simulink model "C_Nonlinear_alg_transform_6T"  (R2016b)
settings: Solver=ode15s  StartTime=0.0  StopTime=100  RelTol=0.01  AbsTol=0.01
libraries: dspinverses x1
settings Model: Creator=Utente  LastModifiedBy=liana
settings SolverCC: MaxOrder=3  MaxConsecutiveMinStep=5  SolverJacobianMethodControl=FullAnalytical  ZeroCrossControl=DisableAll  SolverResetMethod=Robust
settings DataIOCC: SaveState=on
settings OptimizationCC: BlockReduction=off  DefaultParameterBehavior=Inlined  BufferReuse=off

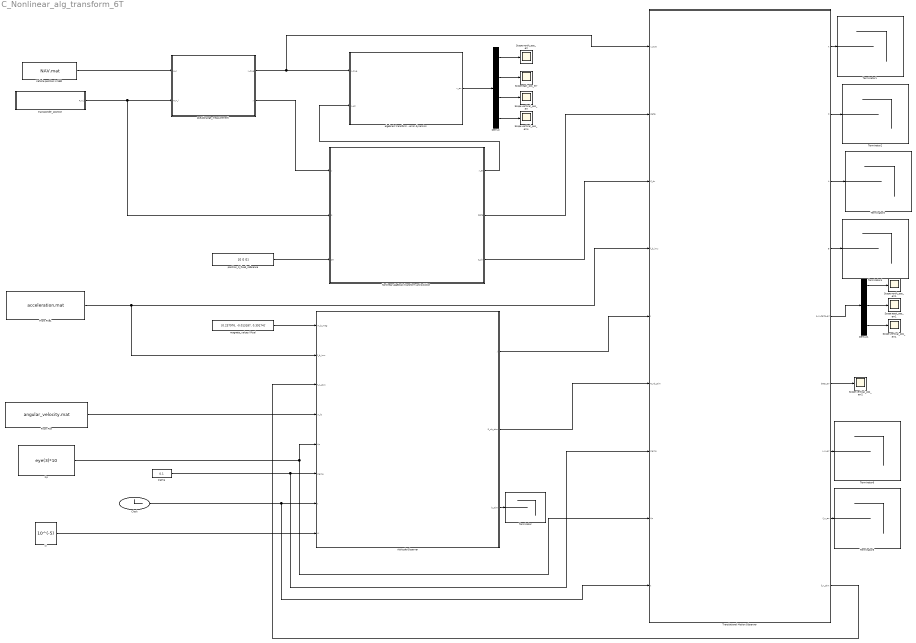
== system C_Nonlinear_alg_transform_6T ==
  Attitude Observer : Subsystem
  Clock : Clock
      settings: Decimation=50
  Demux : Demux
  Demux1 : Demux  Outputs=3
  From File : FromFile  FileName=angular_velocity.mat  SampleTime=0
  From File1 : FromFile  FileName=acceleration.mat  SampleTime=0
  Kp : Constant  Value=eye(3)*10
  Nonlinear algebraic transform and solution : Subsystem
  Scope east_pos_err : Scope
  Scope east_pos_err1 : Scope
  Scope north_pos_err : Scope
  Scope north_pos_err1 : Scope
  Scope vertical_pos_err{,1..2,4} (4 alike) : Scope
  Terminator{,1..6} (7 alike) : Terminator
  Translational Motion Observer : Subsystem
  Vehicle position in NED : FromFile  FileName=NAV.mat
  algebraic transform - error dynamics : Subsystem
  ki : Constant  Value=10^(-5)
  magneto_values (Pisa) : Constant  Value=[0.237976, -0.013187, 0.39174]'
  position_0_fixed_reference : Constant  Value=[0 0 0]
  "pseudorange_measurement " : Subsystem
  sigma : Constant  Value=0.1
  transponder_position : Subsystem
  wires:
  Demux/1 -> Scope north_pos_err/1
  Demux/2 -> Scope east_pos_err/1
  Demux/3 -> Scope vertical_pos_err/1
  Nonlinear algebraic transform and solution/1(x_at) -> algebraic transform - error dynamics/2(x_at)
  Demux/4 -> Scope vertical_pos_err4/1
  position_0_fixed_reference/1 -> Nonlinear algebraic transform and solution/3(p0)
  Nonlinear algebraic transform and solution/2(delta) -> Translational Motion Observer/2(delta)
  Nonlinear algebraic transform and solution/3(C_dx) -> Translational Motion Observer/3(C_dx)
  Vehicle position in NED/1 -> "pseudorange_measurement "/1(p_n)
  "pseudorange_measurement "/2("y ") -> Nonlinear algebraic transform and solution/1(y)
  algebraic transform - error dynamics/1(x_err) -> Demux/1
  transponder_position/1(p_n_i) -> Nonlinear algebraic transform and solution/2(p), "pseudorange_measurement "/2(p_n_i)
  magneto_values (Pisa)/1 -> Attitude Observer/1(m_b_mag)
  Translational Motion Observer/9(f_n_stim) -> Attitude Observer/3(f_n_stim)
  Attitude Observer/1(J) -> Translational Motion Observer/5(J)
  Attitude Observer/2(R_nb_stim) -> Translational Motion Observer/6(R_nb_stim)
  From File1/1 -> Attitude Observer/2(f_b_imu), Translational Motion Observer/4(f_b_imu)
  Kp/1 -> Attitude Observer/5(Kp), Translational Motion Observer/8(Kp)
  sigma/1 -> Translational Motion Observer/7(sigma), Attitude Observer/6(sigma)
  ki/1 -> Attitude Observer/8(Ki)
  Clock/1 -> Translational Motion Observer/9(t), Attitude Observer/7(t)
  From File/1 -> Attitude Observer/4(w_ib)
  Attitude Observer/3(b_stim) -> Terminator/1
  "pseudorange_measurement "/1(x_true) -> Translational Motion Observer/1(x_true), algebraic transform - error dynamics/1(x_true)
  Translational Motion Observer/1(K) -> Terminator1/1
  Translational Motion Observer/2("C ") -> Terminator2/1
  Translational Motion Observer/3(" A") -> Terminator3/1
  Translational Motion Observer/4(B) -> Terminator4/1
  Translational Motion Observer/8(f_n_err) -> Terminator5/1
  Translational Motion Observer/7(v_n_err) -> Terminator6/1
  Demux1/1 -> Scope north_pos_err1/1
  Demux1/2 -> Scope east_pos_err1/1
  Demux1/3 -> Scope vertical_pos_err1/1
  Translational Motion Observer/6(beta_err) -> Scope vertical_pos_err2/1
  Translational Motion Observer/5(p_n_delta_err) -> Demux1/1

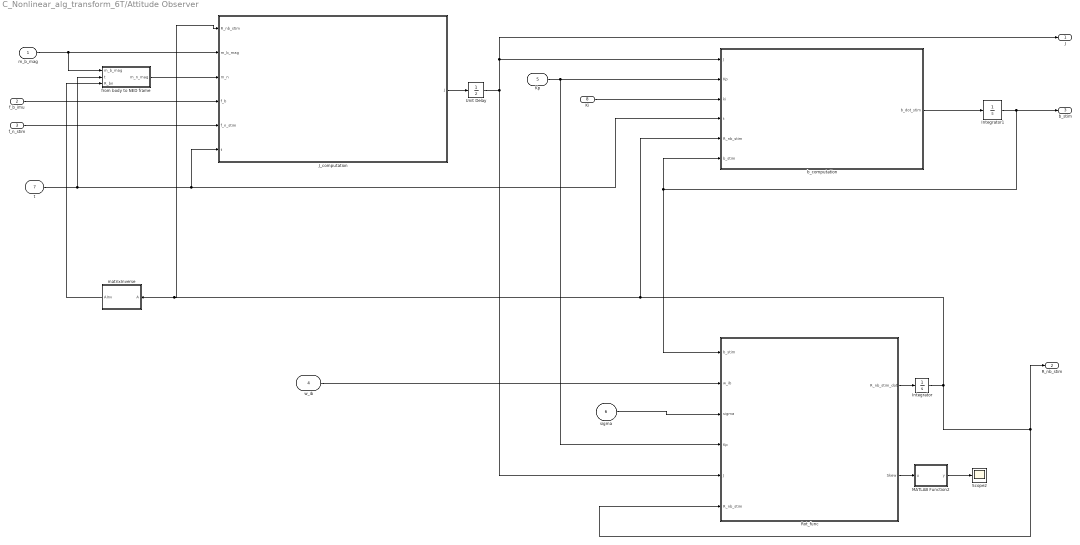
== system C_Nonlinear_alg_transform_6T/Attitude Observer ==
  m_b_mag : Inport
  f_b_imu : Inport  Port=2
  f_n_stim : Inport  Port=3
  w_ib : Inport  Port=4
  Kp : Inport  Port=5
  sigma : Inport  Port=6
  t : Inport  Port=7
  Ki : Inport  Port=8
  Integrator : Integrator  InitialCondition=eye(3)  AbsoluteTolerance=0.0000000001
  Integrator1 : Integrator  InitialCondition=0.02  UpperSaturationLimit=100  LowerSaturationLimit=-100  AbsoluteTolerance=0.0000001
  J_computation : Subsystem
  MATLAB Function2 : MATLAB Function  TreatAsAtomicUnit=on
  Rot_func : MATLAB Function  TreatAsAtomicUnit=on
  Scope2 : Scope
  Unit Delay : UnitDelay  SampleTime=-1
  b_computation : MATLAB Function  TreatAsAtomicUnit=on
  from body to NED frame : MATLAB Function  TreatAsAtomicUnit=on
  matrixInverse : MATLAB Function  TreatAsAtomicUnit=on
  J : Outport
  R_nb_stim : Outport  Port=2
  b_stim : Outport  Port=3
  wires:
  m_b_mag/1 -> from body to NED frame/1(m_b_mag), J_computation/2(m_b_mag)
  from body to NED frame/1(m_n_mag) -> J_computation/3(m_n)
  f_b_imu/1 -> J_computation/4(f_b)
  Kp/1 -> Rot_func/4(Kp), b_computation/2(Kp)
  Ki/1 -> b_computation/3(ki)
  sigma/1 -> Rot_func/3(sigma)
  w_ib/1 -> Rot_func/2(w_ib)
  t/1 -> from body to NED frame/2(t), b_computation/4(t), J_computation/6(t)
  b_computation/1(b_dot_stim) -> Integrator1/1
  matrixInverse/1(AInv) -> from body to NED frame/3(R_bn)
  MATLAB Function2/1(y) -> Scope2/1
  Rot_func/2(Skew) -> MATLAB Function2/1(u)
  Rot_func/1(R_nb_stim_dot) -> Integrator/1
  f_n_stim/1 -> J_computation/5(f_n_stim)
  Integrator/1 -> J_computation/1(R_nb_stim), matrixInverse/1(A), b_computation/5(R_nb_stim), Rot_func/6(R_nb_stim), R_nb_stim/1
  Integrator1/1 -> Rot_func/1(b_stim), b_computation/6(b_stim), b_stim/1
  J_computation/1(J) -> Unit Delay/1
  Unit Delay/1 -> b_computation/1(J), J/1, Rot_func/5(J)

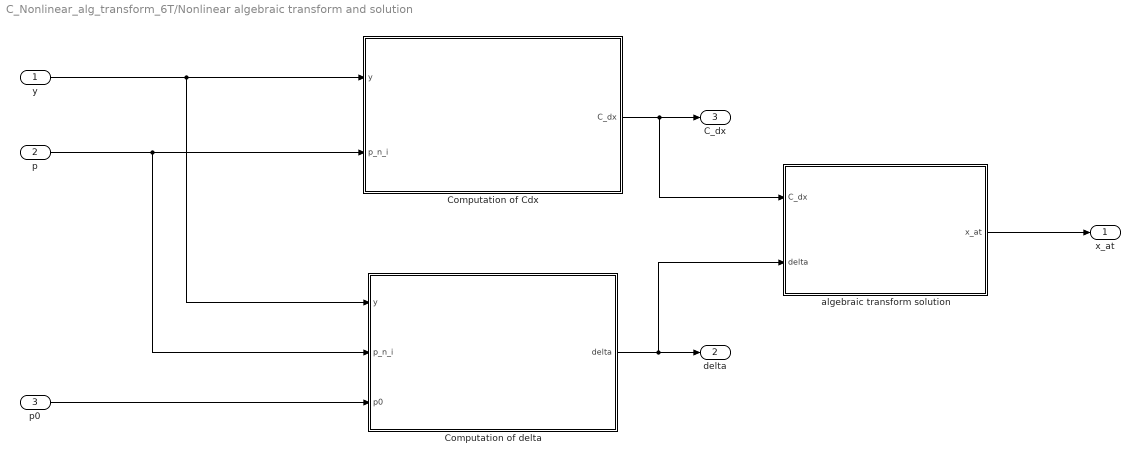
== system C_Nonlinear_alg_transform_6T/Nonlinear algebraic transform and solution ==
  y : Inport
  p : Inport  Port=2
  p0 : Inport  Port=3
  Computation of Cdx : MATLAB Function  TreatAsAtomicUnit=on
  Computation of delta : MATLAB Function  TreatAsAtomicUnit=on
  algebraic transform solution : MATLAB Function  TreatAsAtomicUnit=on
  x_at : Outport
  delta : Outport  Port=2
  C_dx : Outport  Port=3
  wires:
  y/1 -> Computation of delta/1(y), Computation of Cdx/1(y)
  p/1 -> Computation of delta/2(p_n_i), Computation of Cdx/2(p_n_i)
  p0/1 -> Computation of delta/3(p0)
  Computation of delta/1(delta) -> algebraic transform solution/2(delta), delta/1
  Computation of Cdx/1(C_dx) -> algebraic transform solution/1(C_dx), C_dx/1
  algebraic transform solution/1(x_at) -> x_at/1

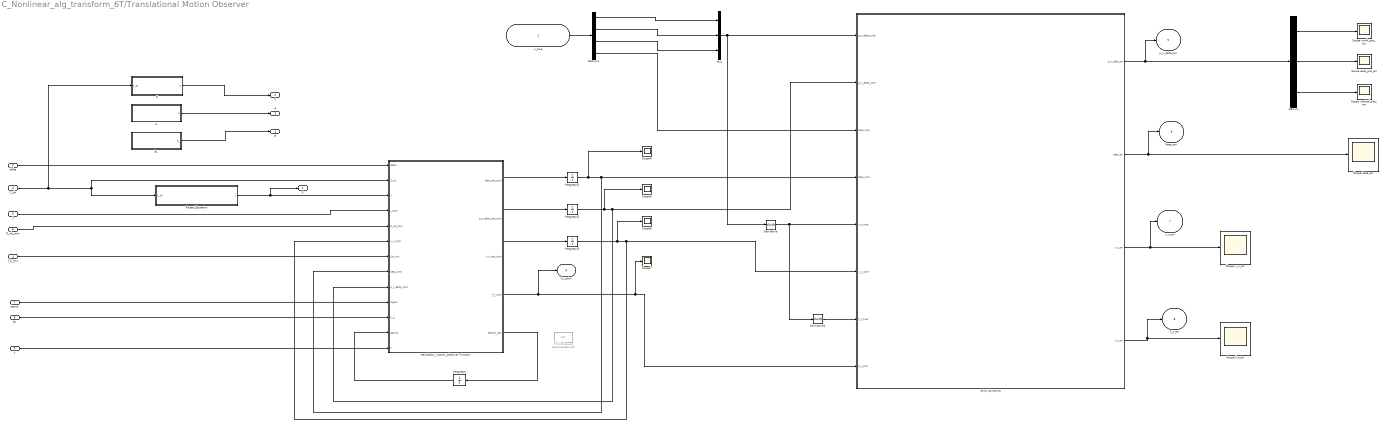
== system C_Nonlinear_alg_transform_6T/Translational Motion Observer ==
  x_true : Inport
  delta : Inport  Port=2
  C_dx : Inport  Port=3
  f_b_imu : Inport  Port=4
  J : Inport  Port=5
  R_nb_stim : Inport  Port=6
  sigma : Inport  Port=7
  Kp : Inport  Port=8
  t : Inport  Port=9
  A : MATLAB Function  TreatAsAtomicUnit=on
  B_ : MATLAB Function  TreatAsAtomicUnit=on
  C : MATLAB Function  TreatAsAtomicUnit=on
  Demux : Demux  Outputs=3
  Demux1 : Demux
  Derivative : Derivative
  Derivative1 : Derivative
  Integrator : Integrator  AbsoluteTolerance=0.01
  Integrator1 : Integrator  InitialCondition=100  AbsoluteTolerance=0.00001
  Integrator2 : Integrator  AbsoluteTolerance=0.01
  Integrator3 : Integrator  AbsoluteTolerance=0.01
  Mux : Mux  Inputs=3
  Riccati_Equation : Subsystem
  Scope beta_err : Scope
  Scope f_n_err : Scope
  Scope v_n_err : Scope
  Scope east_pos_err : Scope
  Scope north_pos_err : Scope
  Scope vertical_pos_err : Scope
  Scope{4..7} (4 alike) : Scope
  To Workspace : ToWorkspace  Commented=on  VariableName=KO  SaveFormat=Timeseries  SampleTime=-1
  error dynamics : MATLAB Function  TreatAsAtomicUnit=on
  translation_motion_observer Function : MATLAB Function  TreatAsAtomicUnit=on
  K : Outport
  "C " : Outport  Port=2
  " A" : Outport  Port=3
  B : Outport  Port=4
  p_n_delta_err : Outport  Port=5
  beta_err : Outport  Port=6
  v_n_err : Outport  Port=7
  f_n_err : Outport  Port=8
  f_n_stim : Outport  Port=9
  wires:
  translation_motion_observer Function/4(f_n_stim) -> f_n_stim/1, Scope7/1, error dynamics/8(f_n_stim)
  translation_motion_observer Function/3(v_n_dot_stim) -> Integrator3/1
  translation_motion_observer Function/2(p_n_delta_dot_stim) -> Integrator2/1
  C_dx/1 -> C/1(C_dx), Riccati_Equation/1(C_dx), translation_motion_observer Function/2(C_dx)
  J/1 -> translation_motion_observer Function/4(J_stim)
  R_nb_stim/1 -> translation_motion_observer Function/5(R_nb_stim)
  delta/1 -> translation_motion_observer Function/1(delta)
  f_b_imu/1 -> translation_motion_observer Function/7(f_b_imu)
  sigma/1 -> translation_motion_observer Function/10(sigma)
  Kp/1 -> translation_motion_observer Function/11(K_p)
  A/1(A) -> " A"/1
  C/1(C) -> "C "/1
  Riccati_Equation/1(K) -> K/1, translation_motion_observer Function/3(K)
  B_/1(B_) -> B/1
  t/1 -> translation_motion_observer Function/13(t)
  Integrator3/1 -> Scope6/1, error dynamics/6(v_n_stim), translation_motion_observer Function/6(v_n_stim)
  translation_motion_observer Function/1(beta_dot_stim) -> Integrator1/1
  Integrator/1 -> translation_motion_observer Function/12(epsilon)
  Integrator1/1 -> Scope4/1, translation_motion_observer Function/8(beta_stim), error dynamics/4(beta_stim)
  translation_motion_observer Function/5(epsilon_dot) -> Integrator/1
  Integrator2/1 -> Scope5/1, error dynamics/2(p_n_delta_stim), translation_motion_observer Function/9(p_n_delta_stim)
  Mux/1 -> Derivative/1, error dynamics/1(p_n_delta_true)
  Demux1/4 -> error dynamics/3(beta_true)
  Derivative1/1 -> error dynamics/7(f_n_true)
  error dynamics/2(beta_err) -> beta_err/1, Scope beta_err/1
  error dynamics/4(f_n_err) -> f_n_err/1, Scope f_n_err/1
  error dynamics/3(v_n_err) -> v_n_err/1, Scope v_n_err/1
  error dynamics/1(p_n_delta_err) -> Demux/1, p_n_delta_err/1
  Demux/1 -> Scope north_pos_err/1
  Demux/2 -> Scope east_pos_err/1
  Demux/3 -> Scope vertical_pos_err/1
  x_true/1 -> Demux1/1
  Demux1/3 -> Mux/3
  Demux1/2 -> Mux/2
  Demux1/1 -> Mux/1
  Derivative/1 -> Derivative1/1, error dynamics/5(v_n_true)

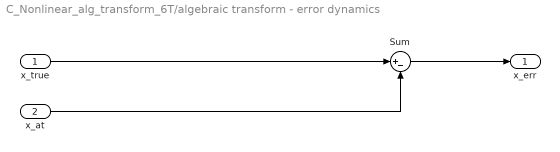
== system C_Nonlinear_alg_transform_6T/algebraic transform - error dynamics ==
  x_true : Inport
  x_at : Inport  Port=2
  Sum : Sum  Inputs=|+-
  x_err : Outport
  wires:
  x_at/1 -> Sum/2
  Sum/1 -> x_err/1
  x_true/1 -> Sum/1

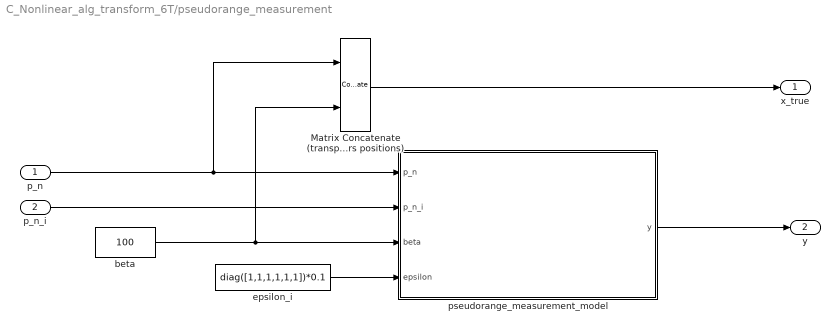
== system C_Nonlinear_alg_transform_6T/pseudorange_measurement  ==
  p_n : Inport
  p_n_i : Inport  Port=2
  Matrix Concatenate (transponders positions) : Concatenate  Mode=Multidimensional array
  beta : Constant  Value=100
  epsilon_i : Constant  Value=diag([1,1,1,1,1,1])*0.1
  pseudorange_measurement_model : MATLAB Function  TreatAsAtomicUnit=on
  x_true : Outport
  "y " : Outport  Port=2
  wires:
  p_n_i/1 -> pseudorange_measurement_model/2(p_n_i)
  pseudorange_measurement_model/1(y) -> "y "/1
  epsilon_i/1 -> pseudorange_measurement_model/4(epsilon)
  beta/1 -> Matrix Concatenate (transponders positions)/2, pseudorange_measurement_model/3(beta)
  p_n/1 -> Matrix Concatenate (transponders positions)/1, pseudorange_measurement_model/1(p_n)
  Matrix Concatenate (transponders positions)/1 -> x_true/1

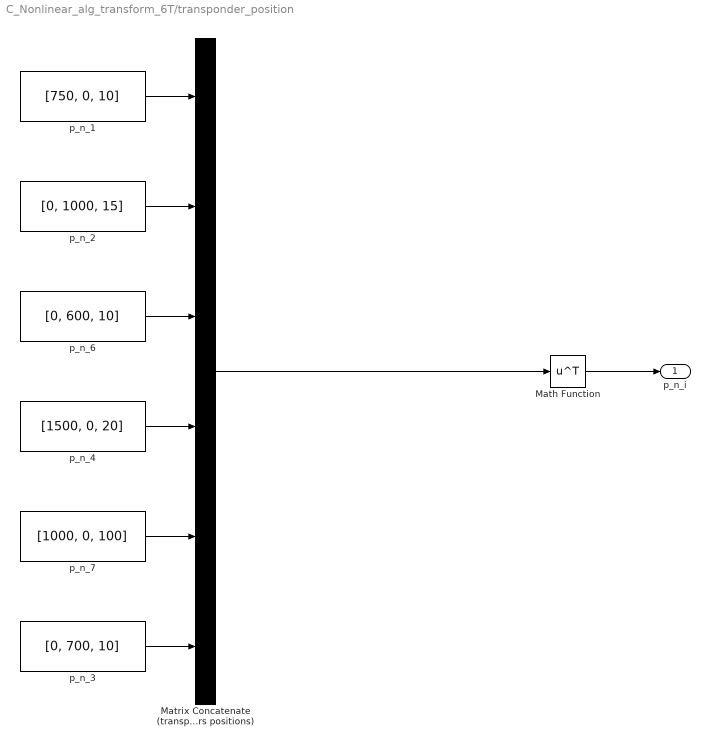
== system C_Nonlinear_alg_transform_6T/transponder_position ==
  Math Function : Math  Operator=transpose  SaturateOnIntegerOverflow=on
  Matrix Concatenate (transponders positions) : Concatenate  NumInputs=6  Mode=Multidimensional array  ConcatenateDimension=2
  p_n_1 : Constant  Value=[750, 0, 10]
  p_n_2 : Constant  Value=[0, 1000, 15]
  p_n_3 : Constant  Value=[0, 700, 10]
  p_n_4 : Constant  Value=[1500, 0, 20]
  p_n_6 : Constant  Value=[0, 600, 10]
  p_n_7 : Constant  Value=[1000, 0, 100]
  p_n_i : Outport
  wires:
  Matrix Concatenate (transponders positions)/1 -> Math Function/1
  p_n_4/1 -> Matrix Concatenate (transponders positions)/4
  p_n_7/1 -> Matrix Concatenate (transponders positions)/5
  p_n_3/1 -> Matrix Concatenate (transponders positions)/6
  Math Function/1 -> p_n_i/1
  p_n_1/1 -> Matrix Concatenate (transponders positions)/1
  p_n_2/1 -> Matrix Concatenate (transponders positions)/2
  p_n_6/1 -> Matrix Concatenate (transponders positions)/3

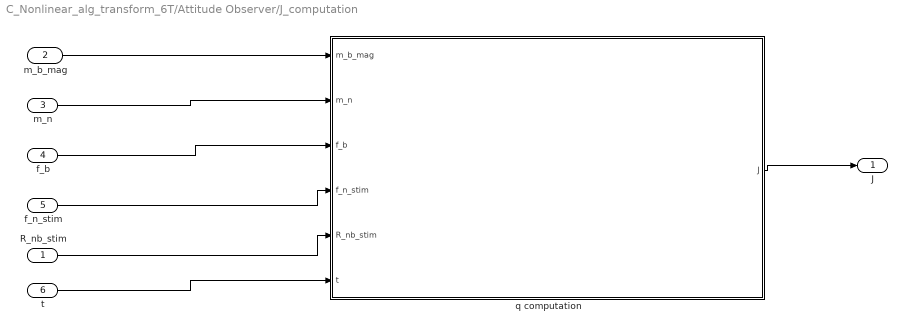
== system C_Nonlinear_alg_transform_6T/Attitude Observer/J_computation ==
  R_nb_stim : Inport
  m_b_mag : Inport  Port=2
  m_n : Inport  Port=3
  f_b : Inport  Port=4
  f_n_stim : Inport  Port=5
  t : Inport  Port=6
  q computation : MATLAB Function  TreatAsAtomicUnit=on
  J : Outport
  wires:
  m_n/1 -> q computation/2(m_n)
  f_n_stim/1 -> q computation/4(f_n_stim)
  m_b_mag/1 -> q computation/1(m_b_mag)
  f_b/1 -> q computation/3(f_b)
  q computation/1(J) -> J/1
  R_nb_stim/1 -> q computation/5(R_nb_stim)
  t/1 -> q computation/6(t)

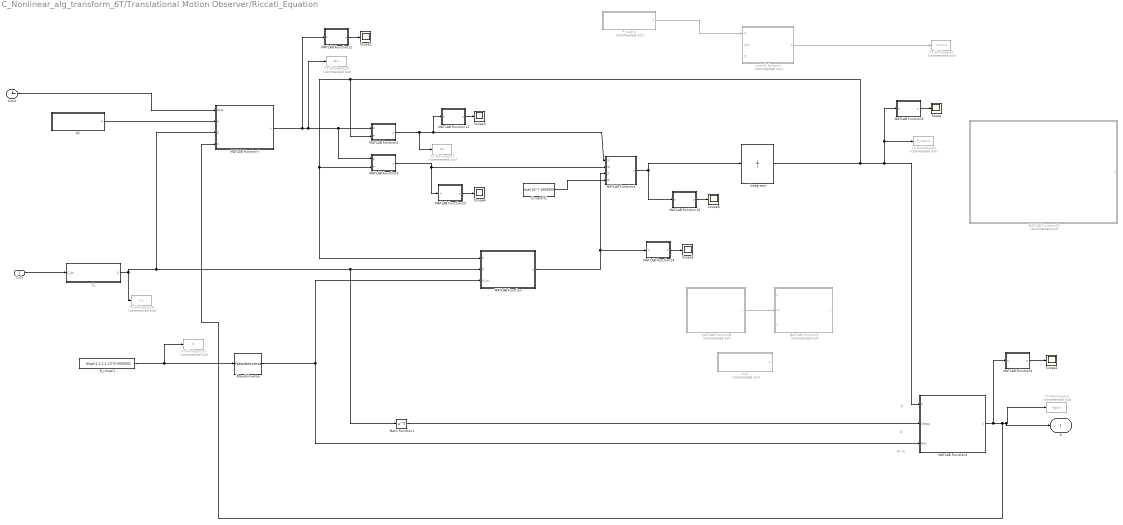
== system C_Nonlinear_alg_transform_6T/Translational Motion Observer/Riccati_Equation ==
  note: R^-1
  note: C'
  note: P
  C_dx : Inport
  A1 : MATLAB Function  TreatAsAtomicUnit=on
  C_ : MATLAB Function  TreatAsAtomicUnit=on
  Clock : Clock
  Integrator : Integrator  InitialCondition=eye(10)*10  AbsoluteTolerance=0.000001
  MATLAB Function : MATLAB Function  TreatAsAtomicUnit=on
  MATLAB Function1 : MATLAB Function  TreatAsAtomicUnit=on
  MATLAB Function10 : MATLAB Function  Commented=on  TreatAsAtomicUnit=on
  MATLAB Function11 : MATLAB Function  TreatAsAtomicUnit=on
  MATLAB Function12 : MATLAB Function  TreatAsAtomicUnit=on
  MATLAB Function13 : MATLAB Function  TreatAsAtomicUnit=on
  MATLAB Function14 : MATLAB Function  TreatAsAtomicUnit=on
  MATLAB Function16 : MATLAB Function  TreatAsAtomicUnit=on
  MATLAB Function2 : MATLAB Function  TreatAsAtomicUnit=on
  MATLAB Function3 : MATLAB Function  TreatAsAtomicUnit=on
  MATLAB Function4 : MATLAB Function  TreatAsAtomicUnit=on
  MATLAB Function5 : MATLAB Function  TreatAsAtomicUnit=on
  MATLAB Function6 : MATLAB Function  TreatAsAtomicUnit=on
  MATLAB Function7 : MATLAB Function  TreatAsAtomicUnit=on
  MATLAB Function8 : MATLAB Function  Commented=on  TreatAsAtomicUnit=on
  MATLAB Function9 : MATLAB Function  Commented=on  TreatAsAtomicUnit=on
  Math Function1 : Math  Operator=transpose  SaturateOnIntegerOverflow=on
  "P_matrix " : MATLAB Function  Commented=on  TreatAsAtomicUnit=on
  Pseudoinverse : dspinverses/Pseudoinverse  wanterr=off  SimulateUsing=Interpreted execution
  Q matrix1 : Constant  Value=eye(10) * 1000000
  R_riccati1 : Constant  Value=diag([1,1,1,1,1])*0.0000001  VectorParams1D=off
  Scope{,1..6} (7 alike) : Scope
  To Workspace1 : ToWorkspace  Commented=on  VariableName=P_matrix  SampleTime=-1
  To Workspace2 : ToWorkspace  Commented=on  VariableName=simout  SaveFormat=Timeseries  SampleTime=-1
  To Workspace3 : ToWorkspace  Commented=on  VariableName=Kgain  SaveFormat=Timeseries  SampleTime=-1
  To Workspace5 : ToWorkspace  Commented=on  VariableName=R  SaveFormat=Timeseries  SampleTime=-1
  To Workspace7 : ToWorkspace  Commented=on  VariableName=PA  SaveFormat=Timeseries  SampleTime=-1
  To Workspace8 : ToWorkspace  Commented=on  VariableName=C_n  SaveFormat=Timeseries  SampleTime=-1
  To Workspace9 : ToWorkspace  Commented=on  VariableName=AKC  SaveFormat=Timeseries  SampleTime=-1
  myC : MATLAB Function  Commented=on  TreatAsAtomicUnit=on
  switch_function : MATLAB Function  Commented=on  TreatAsAtomicUnit=on
  K : Outport
  wires:
  R_riccati1/1 -> Pseudoinverse/1, To Workspace5/1
  Math Function1/1 -> MATLAB Function4/2(Ctrasp)
  MATLAB Function2/1(y) -> To Workspace7/1, MATLAB Function12/1(u), MATLAB Function1/1(X)
  MATLAB Function3/1(y) -> MATLAB Function13/1(u), MATLAB Function1/2(W)
  MATLAB Function/1(y) -> MATLAB Function14/1(u), MATLAB Function1/3(Z)
  MATLAB Function1/1(y) -> Integrator/1, MATLAB Function16/1(u)
  C_dx/1 -> C_/1(C_dx)
  Clock/1 -> MATLAB Function7/1(clock)
  "P_matrix "/1(P) -> switch_function/1(P1)
  switch_function/1(P) -> To Workspace2/1
  Integrator/1 -> MATLAB Function4/1(P), MATLAB Function5/1(u), To Workspace1/1, MATLAB Function2/2(P), MATLAB Function3/2(P), MATLAB Function/1(P)
  MATLAB Function5/1(y) -> Scope/1
  MATLAB Function6/1(y) -> Scope1/1
  MATLAB Function8/1(y) -> MATLAB Function9/2(CK)
  MATLAB Function4/1(y) -> MATLAB Function6/1(u), MATLAB Function7/4(K), K/1, To Workspace3/1
  A1/1(A) -> MATLAB Function7/2(A)
  C_/1(C) -> To Workspace8/1, MATLAB Function7/3(C), Math Function1/1, MATLAB Function/2(C)
  MATLAB Function7/1(y) -> MATLAB Function11/1(u), To Workspace9/1, MATLAB Function3/1(A), MATLAB Function2/1(A)
  MATLAB Function11/1(y) -> Scope2/1
  MATLAB Function12/1(y) -> Scope3/1
  MATLAB Function13/1(y) -> Scope4/1
  MATLAB Function14/1(y) -> Scope5/1
  Pseudoinverse/1 -> MATLAB Function4/3(Rinv), MATLAB Function/3(R_inv)
  MATLAB Function16/1(y) -> Scope6/1
  Q matrix1/1 -> MATLAB Function1/4(Q)

== matlab function C_Nonlinear_alg_transform_6T/Translational Motion Observer/Riccati_Equation/MATLAB Function ==
  data: P input; y output; C input; R_inv input
function y = fcn(P,C,R_inv)

y = - P * C' * R_inv * C * P;

end

== matlab function C_Nonlinear_alg_transform_6T/Attitude Observer/J_computation/q computation ==
  data: m_b_mag input; m_n input; f_b input; f_n_stim input size=3; J output; R_nb_stim input size=[3,3]; t input
function J  = qEfunc(m_b_mag, m_n, f_b, f_n_stim, R_nb_stim, t)

% if t <= 1
%     R_nb_stim = eye(3);
% end

g_n = [0.1 0.1 9.81]';

q1_b = m_b_mag/norm(m_b_mag,2);
q2_b = f_b/norm(g_n,2);

q1_n = m_n/norm(m_n,2);
q2_n = f_n_stim/norm(g_n,2);


E_b = [q1_b, skew(q1_b)*q2_b, (skew(q1_b)*skew(q1_b))*q2_b];
E_n = [q1_n, skew(q1_n)*q2_n, (skew(q1_n)*skew(q1_n))*q2_n];

J = (E_n - R_nb_stim * E_b) * (E_b');

end

== matlab function C_Nonlinear_alg_transform_6T/Translational Motion Observer/Riccati_Equation/MATLAB Function1 ==
  data: X input; y output size=[10,10]; W input; Z input; Q input
function y = fcn(X,W,Z,Q)

y =  X + W + Z + Q;
% y = Z + Q;

end

== matlab function C_Nonlinear_alg_transform_6T/Translational Motion Observer/Riccati_Equation/A1 ==
  data: A output
function A = A()

 A = zeros(10);

A(1:3,5:7) = eye(3);
A(5:7,8:10) = eye(3);
 

% A = eye(10);

end

== matlab function C_Nonlinear_alg_transform_6T/Attitude Observer/b_computation ==
  data: J input; b_dot_stim output size=3; Kp input; ki input; t input; R_nb_stim input; b_stim input
function b_dot_stim  = b_dot_stim_func(J, Kp, ki, t, R_nb_stim, b_stim)


%b_dot_stim = zeros(3 ,1);

% if t <= 1
%     R_nb_stim = eye(3);
% %      b_stim = zeros(3, 1);
% %     
% end

SAT = sat(R_nb_stim)';
PA = pa( SAT * Kp * J);
VEX = vexfunc(PA);
b_dot_stim = Proj(b_stim , -ki * VEX);
% b_dot_stim = Proj(-ki * VEX, 0.5);

end

== matlab function C_Nonlinear_alg_transform_6T/Translational Motion Observer/translation_motion_observer Function ==
  data: delta input; C_dx input; K input; beta_dot_stim output; J_stim input; R_nb_stim input; p_n_delta_dot_stim output; v_n_dot_stim output; f_n_stim output size=[3,1]; v_n_stim input size=3; f_b_imu input size=3; beta_stim input; p_n_delta_stim input size=3; sigma input; K_p input; epsilon_dot output; epsilon input size=3; t input
function [beta_dot_stim,p_n_delta_dot_stim,v_n_dot_stim,f_n_stim,epsilon_dot] =  TMO_func(delta,C_dx,K,J_stim,R_nb_stim, v_n_stim,f_b_imu, beta_stim, p_n_delta_stim,sigma,K_p,epsilon,t)

%obtained by Riccati equation
 K_pp = K(1:3,:); 
 K_beta_p = K(4,:);
 K_v_p = K(5:7,:);
 K_eps_p = K(8:10,:);

% remember to insert a clock to define dimensions of all variables
g_n = [0.1 0.1 9.81]';

if(t == 0) 
    delta_stim = zeros(3, 1);
    delta_diff = zeros(3, 1);
    v_n_stim = zeros(3, 1);
%     beta_stim = 0;
    epsilon = zeros(3,1);
    p_n_delta_stim = zeros(3, 1);
        
end



x_stim = [p_n_delta_stim; beta_stim];
%delta_stim = 2*C_dx*x_stim;
%delta_diff = (delta - delta_stim);



p_n_delta_dot_stim = v_n_stim + K_pp * (delta - 2*C_dx*x_stim);       % eq 14


beta_dot_stim = K_beta_p * (delta - 2*C_dx*x_stim);                       % eq 15

f_n_stim = R_nb_stim * f_b_imu + epsilon ;         % eq 18


v_n_dot_stim  = f_n_stim + g_n + K_v_p*(delta - 2*C_dx*x_stim);         % eq 16


epsilon_dot   = -sigma * K_p * J_stim * f_b_imu + K_eps_p * (delta - 2*C_dx * x_stim); % eq 17

end

== matlab function C_Nonlinear_alg_transform_6T/Nonlinear algebraic transform and solution/Computation of Cdx ==
  data: y input; p_n_i input; C_dx output
function C_dx  = C_dx_func(y,p_n_i)

    % y vector 
    % p matrix has row vectors
    %            (x,y,z) cols 
    %            m-rows are transponders number
    % all variables are in navigation frame oh yeah! baby ;)
    
    [row,col] = size(p_n_i);
    [row_,col_] = size(y);
    
    % m-measure vector
    p_m = p_n_i(row,:); % measure of m-th transponder
    y_m = y(row_);  % m-th pseudorange measure

    m = row; % m is transpoders number
    
    
    p_ = zeros(m-1,3); %row vector, 3 stands for x,y,z
    y_ = zeros(m-1,1);
    
    for i = 1 : 1 : m-1
    
        p_(i,:) = p_m - p_n_i(i,:);
        y_(i) = y(i) - y_m;
        
    end
    
    C_dx = [p_, y_];

end

== matlab function C_Nonlinear_alg_transform_6T/Nonlinear algebraic transform and solution/Computation of delta ==
  data: y input; delta output; p_n_i input; p0 input
function delta   = delta_func(y, p_n_i, p0)

    % y vector 
    % p matrix has row vectors
    %            (x,y,z) cols 
    %            m-rows are the numbers of the transponders
    % all variables are in navigation frame oh yeah! baby ;)
    % z is a col vector of scalars
    
    % we must choose p0 (a block)
    
    [row,col] = size(p_n_i);
    %[row_,col_] = size(y);
    
    p_los = zeros(row,col);
    z = zeros(row,1);   % dim = m x 1
    
    %defining los vector
    for i = 1:1:row
       p_los(i,:) = p_n_i(i,:) - p0';       % dim = m x 3
    end
    
%     p_n_true = p_los;
    
    % p_los = p_los';
    
    for i = 1:1:row
        z(i)= ((y(i)^2) - norm(p_los(i,:))^2); % dim = m x 1
    end
    
%     z = z';
%     
%     delta = zeros(row-1,1);
%     z_m = z(end);
%     
%     for i = 1:1:row-1
%         delta(i) =  (z(i) - z_m); %amm fenito
%     end

    delta = zeros(row-1,1); %dim = (m-1) x 1
    z_m = z(row,1);
    
    for i=1:1:(row-1)
        delta(i,1) = z(i,1) - z_m;
    end

end

== matlab function C_Nonlinear_alg_transform_6T/Translational Motion Observer/Riccati_Equation/MATLAB Function2 ==
  data: A input; y output; P input
function y = fcn(A,P)

y = P * A;

end

== matlab function C_Nonlinear_alg_transform_6T/Translational Motion Observer/Riccati_Equation/MATLAB Function3 ==
  data: A input; y output; P input
function y = fcn(A,P)

y = A' * P;

end

== matlab function C_Nonlinear_alg_transform_6T/Translational Motion Observer/Riccati_Equation/MATLAB Function4 ==
  data: P input; y output; Ctrasp input; Rinv input
function y = fcn(P, Ctrasp, Rinv)

y = P * Ctrasp * Rinv;

end

== matlab function C_Nonlinear_alg_transform_6T/Attitude Observer/Rot_func ==
  data: b_stim input; R_nb_stim_dot output; w_ib input; sigma input; Kp input; J input; R_nb_stim input; Skew output
function [R_nb_stim_dot, Skew] = rot_func(b_stim,w_ib,sigma,Kp,J,R_nb_stim) 

Skew = skew(w_ib - b_stim);

R_nb_stim_dot = R_nb_stim * Skew + sigma * Kp * J;

== matlab function C_Nonlinear_alg_transform_6T/Attitude Observer/MATLAB Function2 ==
  data: u input; y output
function y = fcn(u)

y = norm(u);

== matlab function C_Nonlinear_alg_transform_6T/Translational Motion Observer/Riccati_Equation/C_ ==
  data: C output; C_dx input
function C = C(C_dx)

   row = size(C_dx,1); 

 C1 = zeros(row,6);
 C = [2*C_dx C1];
 

% C1 = zeros(row, 2);
% 
% C = [C_dx C_dx C1];

== matlab function C_Nonlinear_alg_transform_6T/Translational Motion Observer/A ==
  data: A output
function A = A()

 A = zeros(10);

 A(1:3,5:7) = eye(3);
 A(5:7,8:10) = eye(3);
 
end

== matlab function C_Nonlinear_alg_transform_6T/Translational Motion Observer/C ==
  data: C output; C_dx input
function C = Cfunc(C_dx)

   row = size(C_dx,1); 

   C1 = zeros(row,6);

 C = [2*C_dx C1];
 
 
end

== matlab function C_Nonlinear_alg_transform_6T/Translational Motion Observer/B_ ==
  data: B_ output
function B_ = B()

 B_ = zeros(10,3);

 B_(8:10,1:3) = eye(3);
end

== matlab function C_Nonlinear_alg_transform_6T/Translational Motion Observer/Riccati_Equation/P_matrix  ==
  data: P output
function P = P()

P = eye(10);
 
%  P = diag([3 * 10^3,3 * 10^3,3 * 10^3,3 * 10^3,10,10,10,0.01,0.01,0.01]);
 
end

== matlab function C_Nonlinear_alg_transform_6T/pseudorange_measurement /pseudorange_measurement_model ==
  data: p_n input; y output; p_n_i input; beta input; epsilon input
function y = pseudorange_mea_model(p_n, p_n_i, beta, epsilon)

  %  row-vector

  y = zeros(size(p_n_i,1),1);

  for i = 1:1:size(p_n_i,1)

      rho = norm(p_n - (p_n_i(i,:))');  % eq. 7
      
      y(i) = rho + beta + epsilon(i); % eq. 8 

  end
      
end

== matlab function C_Nonlinear_alg_transform_6T/Translational Motion Observer/Riccati_Equation/switch_function ==
  data: P1 input; P output; clock input; P2 input
function P = switch_function(P1, clock, P2)

if clock == 0
    P = P1;
else
    P = P2;
end

end

== matlab function C_Nonlinear_alg_transform_6T/Translational Motion Observer/Riccati_Equation/MATLAB Function5 ==
  data: u input; y output
function y = fcn(u)


y = norm(u);

== matlab function C_Nonlinear_alg_transform_6T/Attitude Observer/from body to NED frame ==
  data: m_b_mag input; t input; R_bn input; m_n_mag output
function m_n_mag = b2n(m_b_mag, t, R_bn)

% m_n_mag and m_b_mag are 3x1

if t==0
    R_bn = eye(3);
end

m_n_mag = R_bn * m_b_mag;

== matlab function C_Nonlinear_alg_transform_6T/Attitude Observer/matrixInverse ==
  data: A input; AInv output
function AInv  = matrixInverse(A)

% inverse by singular value decomposition


[n,m] = size(A);

% U = zeros(n,n);
% V = zeros(n,n);
% S = zeros(n,n);

[U,S,V] = svd(A);

pos = 0;

% maximun admissible condition number
csi = 10^3;

for i=n:-1:1
    if( S(1,1)/S(i,i) > csi)
        S(i,i) = 0;
        pos = i; % keeps the last eliminated singular value
    end
end

tempS = S(1:pos-1,1:pos-1); %take the non-zero set
tempS = inv(tempS);
S(1:pos-1,1:pos-1) = tempS(1:pos-1,1:pos-1); % now S is the inverse matrix
AInv = V * S * U';

end

== matlab function C_Nonlinear_alg_transform_6T/Translational Motion Observer/Riccati_Equation/MATLAB Function6 ==
  data: u input; y output
function y = fcn(u)

y = norm(u);

== matlab function C_Nonlinear_alg_transform_6T/Translational Motion Observer/Riccati_Equation/MATLAB Function7 ==
  data: clock input; y output; A input; C input; K input
function y = fcn(clock, A, C, K)

% if clock <= 20
    y = A;
% else
%     y = A - K*C;
% % end
end

== matlab function C_Nonlinear_alg_transform_6T/Translational Motion Observer/Riccati_Equation/MATLAB Function8 ==
  data: y output
function y = myPlacement()

C =  1000*   [ -1.5000    1.2000         0    0.3000         0         0         0         0  0 0;
         0   -0.8000   -0.0100    0.8001         0         0         0         0    0 0;
   -3.0000   -0.8000   -0.0400    2.4059         0         0         0         0    0 0;
   -3.0000    1.2000   -0.0200    1.8001         0         0         0         0    0 0;
   -1.5000   -0.8000   -0.0300    1.3003         0         0         0         0    0 0];



K = [    10     0     0     0     0;
     0    10     0     0     0;
     0     0    10     0     0;
     0     0     0    10     0;
     0     0     0     0    10;
    10     0     0     0     0;
     0    10     0     0     0;
     0     0    10     0     0;
     0     0     0    10     0;
     0     0     0     0    10];
 
 
 y = K * C;
   
   

end

== matlab function C_Nonlinear_alg_transform_6T/Translational Motion Observer/Riccati_Equation/MATLAB Function9 ==
  data: y output; A input; CK input; t input
function y = oneFun(A, CK, t)

% if t <= 1
    y = A - CK;
% else
%     y = A;

   

end

== matlab function C_Nonlinear_alg_transform_6T/Translational Motion Observer/Riccati_Equation/MATLAB Function10 ==
  data: y output
function y = myGain()

Gain = 1000 * [-1.0308    0.2080   -2.1181   -1.7236   -1.1219;
    1.5540   -0.9782   -1.4402    1.6629   -1.3249;
    1.0278   -2.1284    0.2466   -2.0553   -0.4035;
   -0.1547    0.3620   -0.0435    0.2578   -0.0733;
   -0.0200   -0.3758   -0.8435    0.1880    0.3340;
   -0.6041    0.2009   -0.0138   -0.5953    0.4901;
    0.1845   -0.2811    0.4856    0.3175    0.7418;
   -0.0018    0.0037   -0.0011    0.0037    0.0006;
    0.0004   -0.0011    0.0003   -0.0012    0.0001;
    0.0026   -0.0054    0.0013   -0.0052   -0.0005]

y = Gain;

== matlab function C_Nonlinear_alg_transform_6T/Translational Motion Observer/Riccati_Equation/myC ==
  data: C output
function C = myC()
% 
% C = 1000 * [  -1.5000    1.2000         0    0.3000         0         0         0         0         0   0;
%          0   -0.8000   -0.0100    0.8001         0         0         0         0         0  0;
%    -3.0000   -0.8000   -0.0400    2.4059         0         0         0         0         0  0;
%    -3.0000    1.2000   -0.0200    1.8001         0         0         0         0         0  0;
%    -1.5000   -0.8000   -0.0300    1.3003         0         0         0         0         0  0];
% 
%  
C = zeros(6,10);
C(1:6,1:6) = eye(6);
C(1:3,7:9) = eye(3);
C(4:6,7:9) = eye(3);
end

== matlab function C_Nonlinear_alg_transform_6T/Translational Motion Observer/Riccati_Equation/MATLAB Function11 ==
  data: u input; y output
function y = fcn(u)

y = norm(u);

== matlab function C_Nonlinear_alg_transform_6T/Translational Motion Observer/Riccati_Equation/MATLAB Function12 ==
  data: u input; y output
function y = fcn(u)

y = norm(u(1:8,1:8));

== matlab function C_Nonlinear_alg_transform_6T/Translational Motion Observer/Riccati_Equation/MATLAB Function13 ==
  data: u input; y output
function y = fcn(u)

y = norm(u);

== matlab function C_Nonlinear_alg_transform_6T/Translational Motion Observer/Riccati_Equation/MATLAB Function14 ==
  data: u input; y output
function y = fcn(u)

y = norm(u);

== matlab function C_Nonlinear_alg_transform_6T/Translational Motion Observer/Riccati_Equation/MATLAB Function16 ==
  data: u input; y output
function y = fcn(u)

y = norm(u);

== matlab function C_Nonlinear_alg_transform_6T/Translational Motion Observer/error dynamics ==
  data: p_n_delta_true input; p_n_delta_err output size=[3,1]; p_n_delta_stim input; beta_true input; beta_stim input; beta_err output; v_n_true input; v_n_stim input; f_n_true input; f_n_stim input; v_n_err output; f_n_err output
function [p_n_delta_err, beta_err, v_n_err, f_n_err] = errDyn(p_n_delta_true, p_n_delta_stim, beta_true, beta_stim, v_n_true, v_n_stim, f_n_true, f_n_stim)


p_n_delta_err = p_n_delta_true - p_n_delta_stim;

beta_err = beta_true - beta_stim;

v_n_err = v_n_true - v_n_stim;

f_n_err = f_n_true - f_n_stim;

end

== matlab function C_Nonlinear_alg_transform_6T/Nonlinear algebraic transform and solution/algebraic transform solution ==
  data: C_dx input; x_at output; delta input
function x_at = solAT(C_dx, delta)

% this solution is described in the Appendix
% that is correct only for m >= 5

pC_dx = pinv(C_dx);

x_at = pC_dx * (delta / 2);

end
